simulink model "SIM_NARENDRA_1_METODO_DIFERENCIAL_RECURSIVO_T2_2"  (R2015a)
settings: Solver=ode3  StartTime=0.0  StopTime=16  FixedStep=1e-4  RelTol=1e-3
settings Model: Creator=user  LastModifiedBy=user

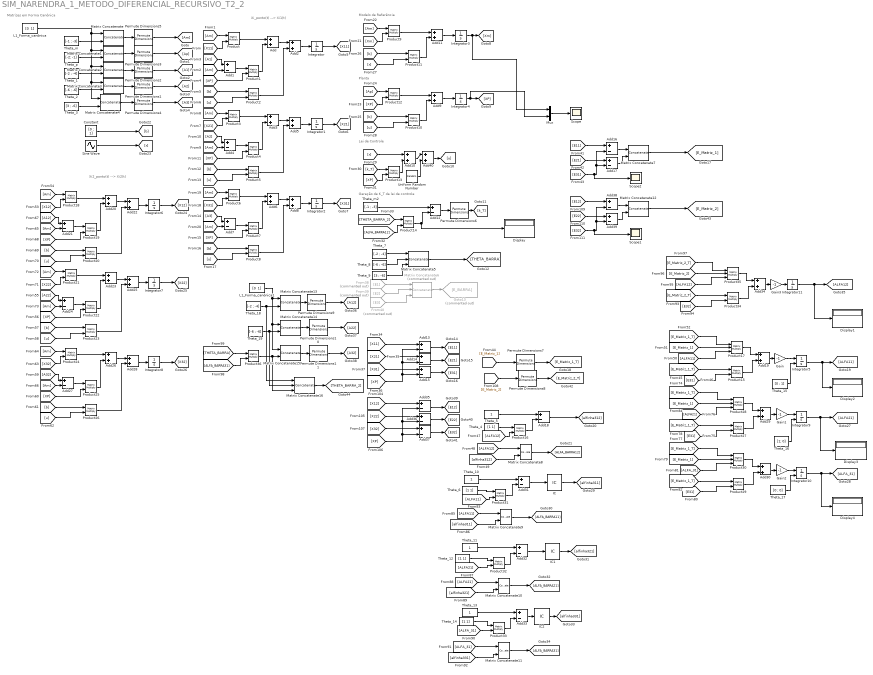
== system SIM_NARENDRA_1_METODO_DIFERENCIAL_RECURSIVO_T2_2 ==
  note: Geração de K_T da lei de controle
  note: Lei de Controle
  note: Planta
  note: Modelo de Referência
  note: Matrizes em Forma Canônica
  note: Xi_ponto(t) --> Xi1(t)
  note: Xi2_ponto(t) --> Xi2(t)
  Add{,2..3,5..6,8..11,19..20,22..23,25..26,28..30,34,40} (20 alike) : Sum
  Add{1,4,7,12..18,21,24,27,31..33,35..39} (21 alike) : Sum  Inputs=+-
  Constant : Constant  Value=[0 ; 1]
  Display{,1..4} (5 alike) : Display
  From38 : From  Commented=on  GotoTag=E1
  From39 : From  Commented=on  GotoTag=E2
  From40 : From  Commented=on  GotoTag=E3
  Gain{,1..3} (4 alike) : Gain  Gain=-1
  Goto13 : Goto  Commented=on  GotoTag=E_BARRA
  IC : InitialCondition
  IC1 : InitialCondition  Value=0
  IC2 : InitialCondition  Value=0.5
  Integrator : Integrator  InitialCondition=[2 2]
  Integrator1 : Integrator  InitialCondition=[1 0]
  Integrator10 : Integrator  InitialConditionSource=external
  Integrator11 : Integrator
  Integrator2 : Integrator  InitialCondition=[0 0]
  Integrator3 : Integrator
  Integrator4 : Integrator  InitialCondition=[0.01 0.02]
  Integrator5 : Integrator  InitialConditionSource=external
  Integrator6 : Integrator  InitialCondition=[2 2]
  Integrator7 : Integrator  InitialCondition=[1 0]
  Integrator8 : Integrator  InitialCondition=[0 0]
  Integrator9 : Integrator  InitialConditionSource=external
  L1_Forma_canônica : Constant  Value="[0  1]"
  L1_Forma_canônica1 : Constant  Value="[0  1]"
  Matrix Concatenate{,1..4,7,12..15} (10 alike) : Concatenate  Mode=Multidimensional array  ConcatenateDimension=2
  Matrix Concatenate{8..11} (4 alike) : Concatenate
  Matrix Concatenate16 : Concatenate  NumInputs=3  Mode=Multidimensional array  ConcatenateDimension=2
  Matrix Concatenate5 : Concatenate  NumInputs=3  Mode=Multidimensional array  ConcatenateDimension=2
  Matrix Concatenate6 : Concatenate  Commented=on  NumInputs=3  Mode=Multidimensional array  ConcatenateDimension=2
  Mux : Mux  Inputs=2
  Permute Dimensions{1..11} (11 alike) : PermuteDimensions
  Product{,1..16,18..27,29,31..34,36} (33 alike) : Product  Multiplication=Matrix(*)
  Product{17,28,30,35} (4 alike) : Product  Inputs=3  Multiplication=Matrix(*)
  Scope : Scope
      settings: YMin=-0.5  YMax=10.5
  Scope1 : Scope
      settings: YMax=35
  Scope2 : Scope
      settings: YMax=55  SaveName=ScopeData2
  Sine Wave : Sin  Bias=10  Frequency=2  SampleTime=0
  Theta_1 : Constant  Value=[-2 ; -4]
  Theta_{5,10..11,13} (4 alike) : Constant
  Theta_{4,6,12,14} (4 alike) : Constant  Value=[1 1]  VectorParams1D=off
  Theta_15 : Constant  Value=[0 ; 1]  VectorParams1D=off
  Theta_16 : Constant  Value=[1; 0]  VectorParams1D=off
  Theta_17 : Constant  Value=[0 ; 0]  VectorParams1D=off
  Theta_18 : Constant  Value=[-2 ; -4]
  Theta_19 : Constant  Value=[-6 ; -6]
  Theta_2 : Constant  Value=[-6 ; -6]
  Theta_3 : Constant  Value=[3 ; -6]
  Theta_7 : Constant  Value=[-2 ; -4]
  Theta_8 : Constant  Value=[-6 ; -6]
  Theta_9 : Constant  Value=[3 ; -6]
  Theta_m : Constant  Value=[-1 ; -3]
  Theta_m2 : Constant  Value=[-1 ; -3]
  Theta_p : Constant  Value=[-2; -1]
  Uniform Random Number : UniformRandomNumber
  wires:
  Theta_m/1 -> Matrix Concatenate/2
  L1_Forma_canônica/1 -> Matrix Concatenate4/1, Matrix Concatenate3/1, Matrix Concatenate2/1, Matrix Concatenate1/1, Matrix Concatenate/1
  Theta_p/1 -> Matrix Concatenate1/2
  Theta_1/1 -> Matrix Concatenate2/2
  Theta_2/1 -> Matrix Concatenate3/2
  Theta_3/1 -> Matrix Concatenate4/2
  Matrix Concatenate/1 -> Permute Dimensions5/1
  Matrix Concatenate1/1 -> Permute Dimensions3/1
  Matrix Concatenate2/1 -> Permute Dimensions2/1
  Matrix Concatenate3/1 -> Permute Dimensions1/1
  Matrix Concatenate4/1 -> Permute Dimensions4/1
  Permute Dimensions4/1 -> [A3]
  Permute Dimensions1/1 -> [A2]
  Permute Dimensions2/1 -> [A1]
  Permute Dimensions3/1 -> [Ap]
  Permute Dimensions5/1 -> [Am]
  [Am] -> Product/1
  [X11] -> Product/2
  Product/1 -> Add/1
  Product1/1 -> Add/2
  Add1/1 -> Product1/1
  [Am] -> Add1/2
  [A1] -> Add1/1
  [XP] -> Product1/2
  Add/1 -> Add2/1
  Product2/1 -> Add2/2
  [b] -> Product2/1
  [u] -> Product2/2
  Add2/1 -> Integrator/1
  Integrator/1 -> [X11]
  [Am] -> Product3/1
  [X21] -> Product3/2
  Product3/1 -> Add3/1
  Product4/1 -> Add3/2
  Add4/1 -> Product4/1
  [Am] -> Add4/2
  [A2] -> Add4/1
  [XP] -> Product4/2
  Add3/1 -> Add5/1
  Product5/1 -> Add5/2
  [b] -> Product5/1
  [u] -> Product5/2
  Add5/1 -> Integrator1/1
  Integrator1/1 -> [X21]
  [X31] -> Product6/2
  Product6/1 -> Add6/1
  Product7/1 -> Add6/2
  Add7/1 -> Product7/1
  [Am] -> Add7/2
  [A3] -> Add7/1
  [XP] -> Product7/2
  Add6/1 -> Add8/1
  Product8/1 -> Add8/2
  [b] -> Product8/1
  [u] -> Product8/2
  Add8/1 -> Integrator2/1
  Integrator2/1 -> [X31]
  [Am] -> Product6/1
  [Xm] -> Product9/2
  Product9/1 -> Add11/1
  Product11/1 -> Add11/2
  [b] -> Product11/1
  [r] -> Product11/2
  Add11/1 -> Integrator3/1
  [Am] -> Product9/1
  [XP] -> Product12/2
  Product12/1 -> Add9/1
  Product10/1 -> Add9/2
  [b] -> Product10/1
  [u] -> Product10/2
  Add9/1 -> Integrator4/1
  Integrator4/1 -> Mux/2, [XP]
  [Ap] -> Product12/1
  [k_T] -> Product13/1
  [XP] -> Product13/2
  Product13/1 -> Add10/2
  [r] -> Add10/1
  Permute Dimensions6/1 -> [k_T]
  [THETA_BARRA_2] -> Product14/1
  [ALFA_BARRA12] -> Product14/2
  Theta_m2/1 -> Add12/1
  Product14/1 -> Display/1, Add12/2
  Add12/1 -> Permute Dimensions6/1
  Theta_7/1 -> Matrix Concatenate5/1
  Theta_8/1 -> Matrix Concatenate5/2
  Theta_9/1 -> Matrix Concatenate5/3
  Matrix Concatenate5/1 -> [THETA_BARRA]
  [X11] -> Add13/1
  [XP] -> Add15/2, Add14/2, Add13/2
  [X21] -> Add14/1
  [X31] -> Add15/1
  Add13/1 -> [E11]
  Add14/1 -> [E21]
  Add15/1 -> [E31]
  Matrix Concatenate6/1 -> Goto13/1
  From38/1 -> Matrix Concatenate6/1
  From39/1 -> Matrix Concatenate6/2
  From40/1 -> Matrix Concatenate6/3
  [E31] -> Scope2/1, Add17/2, Add16/2
  [E11] -> Add16/1
  [E21] -> Add17/1
  Add17/1 -> Matrix Concatenate7/2
  Add16/1 -> Matrix Concatenate7/1
  [E_Matriz_1] -> Permute Dimensions7/1
  [E_Matriz_1_T] -> Product15/1
  Theta_5/1 -> Add18/1
  Product16/1 -> Add18/2
  [ALFA12] -> Matrix Concatenate8/1
  [alfinha312] -> Matrix Concatenate8/2
  Matrix Concatenate8/1 -> [ALFA_BARRA12]
  Constant/1 -> [b]
  Sine Wave/1 -> [r]
  Matrix Concatenate7/1 -> [E_Matriz_1]
  Integrator3/1 -> Mux/1, [Xm]
  Mux/1 -> Scope/1
  Product15/1 -> Add19/2
  Add18/1 -> [alfinha312]
  [E31] -> Product15/2
  Permute Dimensions7/1 -> [E_Matriz_1_T]
  [ALFA11] -> Product17/3
  Product17/1 -> Add19/1
  Add19/1 -> Gain/1
  Gain/1 -> Integrator5/1
  [E_Matriz_1] -> Product17/2
  [E_Matriz_1_T] -> Product17/1
  [Am] -> Product18/1
  [X12] -> Product18/2
  Product18/1 -> Add20/1
  Product19/1 -> Add20/2
  Add21/1 -> Product19/1
  [Am] -> Add21/2
  [A12] -> Add21/1
  [XP] -> Product19/2
  Add20/1 -> Add22/1
  Product20/1 -> Add22/2
  [b] -> Product20/1
  [u] -> Product20/2
  Add22/1 -> Integrator6/1
  Integrator6/1 -> [X12]
  [Am] -> Product21/1
  [X22] -> Product21/2
  Product21/1 -> Add23/1
  Product22/1 -> Add23/2
  Add24/1 -> Product22/1
  [Am] -> Add24/2
  [A22] -> Add24/1
  [XP] -> Product22/2
  Add23/1 -> Add25/1
  Product23/1 -> Add25/2
  [b] -> Product23/1
  [u] -> Product23/2
  Add25/1 -> Integrator7/1
  Integrator7/1 -> [X22]
  [X32] -> Product24/2
  Product24/1 -> Add26/1
  Product25/1 -> Add26/2
  Add27/1 -> Product25/1
  [Am] -> Add27/2
  [A32] -> Add27/1
  [XP] -> Product25/2
  Add26/1 -> Add28/1
  Product26/1 -> Add28/2
  [b] -> Product26/1
  [u] -> Product26/2
  Add28/1 -> Integrator8/1
  Integrator8/1 -> [X32]
  [Am] -> Product24/1
  [E_Matriz_1_T] -> Product27/1
  Product27/1 -> Add29/2
  [E31] -> Product27/2
  [ALFA21] -> Product28/3
  Product28/1 -> Add29/1
  Add29/1 -> Gain1/1
  Integrator9/1 -> Display3/1, [ALFA21]
  Gain1/1 -> Integrator9/1
  [E_Matriz_1] -> Product28/2
  [E_Matriz_1_T] -> Product28/1
  [E_Matriz_1_T] -> Product29/1
  Product29/1 -> Add30/2
  [E31] -> Product29/2
  [ALFA_31] -> Product30/3
  Product30/1 -> Add30/1
  Add30/1 -> Gain2/1
  Integrator10/1 -> Display4/1, [ALFA_31]
  Gain2/1 -> Integrator10/1
  [E_Matriz_1] -> Product30/2
  [E_Matriz_1_T] -> Product30/1
  Theta_10/1 -> Add31/1
  Product31/1 -> Add31/2
  [ALFA11] -> Matrix Concatenate9/1
  [alfinha311] -> Matrix Concatenate9/2
  Matrix Concatenate9/1 -> [ALFA_BARRA11]
  Add31/1 -> IC/1
  Theta_12/1 -> Product32/1
  Theta_11/1 -> Add32/1
  Product32/1 -> Add32/2
  [ALFA21] -> Matrix Concatenate10/1
  [alfinha321] -> Matrix Concatenate10/2
  Matrix Concatenate10/1 -> [ALFA_BARRA21]
  Add32/1 -> IC1/1
  [ALFA_31] -> Product33/2
  Theta_13/1 -> Add33/1
  Product33/1 -> Add33/2
  [ALFA_31] -> Matrix Concatenate11/1
  [alfinha331] -> Matrix Concatenate11/2
  Matrix Concatenate11/1 -> [ALFA_BARRA31]
  Add33/1 -> IC2/1
  [E_Matriz_2_T] -> Product34/1
  Product34/1 -> Add34/2
  [E32] -> Product34/2
  [ALFA12] -> Product35/3
  Product35/1 -> Add34/1
  Add34/1 -> Gain3/1
  Integrator11/1 -> Display1/1, [ALFA12]
  Gain3/1 -> Integrator11/1
  [E_Matriz_2] -> Product35/2
  [E_Matriz_2_T] -> Product35/1
  [X12] -> Add35/1
  [XP] -> Add35/2, Add36/2, Add37/2
  [X22] -> Add36/1
  [X32] -> Add37/1
  Add35/1 -> [E12]
  Add36/1 -> [E22]
  Add37/1 -> [E32]
  [E_Matriz_2] -> Permute Dimensions8/1
  Permute Dimensions8/1 -> [E_Matriz_2_T]
  [E32] -> Add38/2, Add39/2, Scope1/1
  [E12] -> Add38/1
  [E22] -> Add39/1
  Add39/1 -> Matrix Concatenate12/2
  Add38/1 -> Matrix Concatenate12/1
  Matrix Concatenate12/1 -> [E_Matriz_2]
  Matrix Concatenate15/1 -> Permute Dimensions11/1
  Matrix Concatenate13/1 -> Permute Dimensions9/1
  Theta_18/1 -> Matrix Concatenate16/1, Matrix Concatenate13/2
  Theta_19/1 -> Matrix Concatenate16/2, Matrix Concatenate14/2
  Product36/1 -> Matrix Concatenate16/3, Matrix Concatenate15/2
  L1_Forma_canônica1/1 -> Matrix Concatenate15/1, Matrix Concatenate14/1, Matrix Concatenate13/1
  Matrix Concatenate16/1 -> [THETA_BARRA_2]
  Integrator5/1 -> Display2/1, [ALFA11]
  IC/1 -> [alfinha311]
  IC1/1 -> [alfinha321]
  IC2/1 -> [alfinha331]
  Theta_17/1 -> Integrator10/2
  Theta_16/1 -> Integrator9/2
  Theta_15/1 -> Integrator5/2
  Theta_6/1 -> Product31/1
  [ALFA11] -> Product31/2
  [ALFA21] -> Product32/2
  Theta_14/1 -> Product33/1
  Theta_4/1 -> Product16/1
  [ALFA12] -> Product16/2
  Add40/1 -> [u]
  Add10/1 -> Add40/1
  Uniform Random Number/1 -> Add40/2
  Matrix Concatenate14/1 -> Permute Dimensions10/1
  Permute Dimensions9/1 -> [A12]
  Permute Dimensions10/1 -> [A22]
  Permute Dimensions11/1 -> [A32]
  [THETA_BARRA] -> Product36/1
  [ALFA_BARRA31] -> Product36/2
